simulink model "Ex_1_8"  (R2020a)
settings: Solver=VariableStepAuto  StartTime=0.0  StopTime=100  RelTol=1e-3
libraries: simulink x1
settings Model: Creator=dimit  LastModifiedBy=dimit

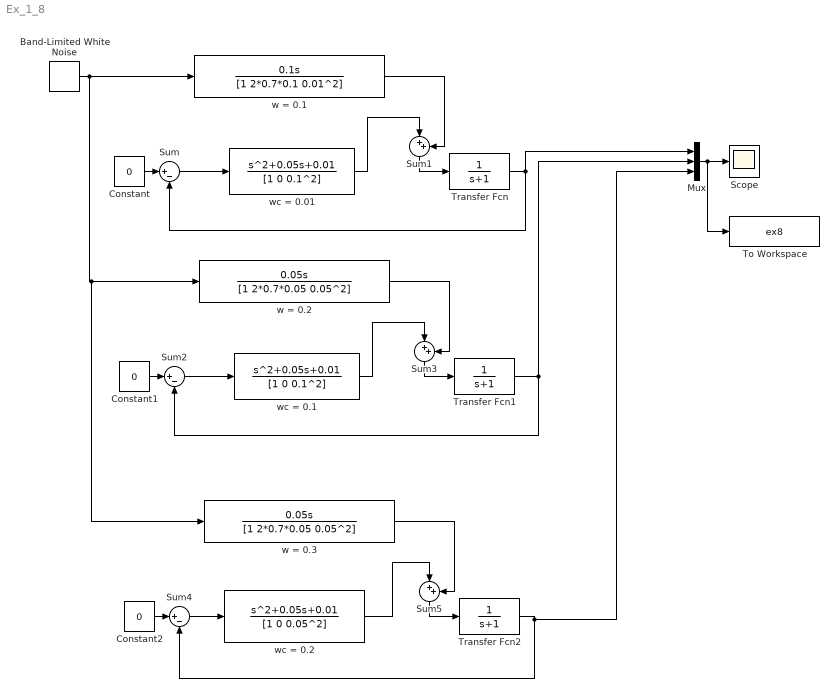
== system Ex_1_8 ==
  Band-Limited White Noise : simulink/Sources/Band-Limited White Noise  Cov=[25]  Ts=0.1  seed=[23341]
  Constant : Constant  Value=0
  Constant1 : Constant  Value=0
  Constant2 : Constant  Value=0
  Mux : Mux  Inputs=3
  Scope : Scope
  Sum : Sum  Inputs=|+-
  Sum1 : Sum  Inputs=|++
  Sum2 : Sum  Inputs=|+-
  Sum3 : Sum  Inputs=|++
  Sum4 : Sum  Inputs=|+-
  Sum5 : Sum  Inputs=|++
  To Workspace : ToWorkspace  VariableName=ex8  SaveFormat=Timeseries  SampleTime=-1
  Transfer Fcn : TransferFcn  Denominator=[1 1]
  Transfer Fcn1 : TransferFcn  Denominator=[1 1]
  Transfer Fcn2 : TransferFcn  Denominator=[1 1]
  w = 0.1 : TransferFcn  Numerator=[0.1 0]  Denominator=[1 2*0.7*0.1 0.01^2]
  w = 0.2 : TransferFcn  Numerator=[0.05 0]  Denominator=[1 2*0.7*0.05 0.05^2]
  w = 0.3 : TransferFcn  Numerator=[0.05 0]  Denominator=[1 2*0.7*0.05 0.05^2]
  wc = 0.01 : TransferFcn  Numerator=[1 0.05 0.01]  Denominator=[1 0 0.1^2]
  wc = 0.1 : TransferFcn  Numerator=[1 0.05 0.01]  Denominator=[1 0 0.1^2]
  wc = 0.2 : TransferFcn  Numerator=[1 0.05 0.01]  Denominator=[1 0 0.05^2]
  wires:
  Sum/1 -> wc = 0.01/1
  Constant/1 -> Sum/1
  wc = 0.01/1 -> Sum1/1
  w = 0.1/1 -> Sum1/2
  Sum1/1 -> Transfer Fcn/1
  Transfer Fcn/1 -> Mux/1, Sum/2
  w = 0.2/1 -> Sum3/2
  Sum2/1 -> wc = 0.1/1
  Sum3/1 -> Transfer Fcn1/1
  Transfer Fcn1/1 -> Mux/2, Sum2/2
  Constant1/1 -> Sum2/1
  wc = 0.1/1 -> Sum3/1
  Band-Limited White Noise/1 -> w = 0.3/1, w = 0.2/1, w = 0.1/1
  Constant2/1 -> Sum4/1
  wc = 0.2/1 -> Sum5/1
  w = 0.3/1 -> Sum5/2
  Sum5/1 -> Transfer Fcn2/1
  Sum4/1 -> wc = 0.2/1
  Transfer Fcn2/1 -> Mux/3, Sum4/2
  Mux/1 -> To Workspace/1, Scope/1
